simulink model "PASTd_2024"  (R2024b)
settings: Solver=VariableStepAuto  StartTime=0.0  StopTime=20  RelTol=1e-3
model workspace: external: MATLAB File PASTd_2024_saveas.m (data not in the file)
values from neighbouring files (symbols this model uses):
  B_table = cmap(:,3)'    [run.m]
  d0 = 0.01    [run.m]
  G_table = cmap(:,2)'    [run.m]
  R_table = cmap(:,1)'    [run.m]
  w0 = ones(l*w,1)    [run.m]
undefined symbols (not defined in the file or in its folder): hot, intensity_max, intensity_min, l, lower_raw, magnitude, upper_raw, w
libraries: dsparch4 x9, matrix_library x1, dspsrcs4 x1
settings Model: PacingRate=10  Creator=yingwan  LastModifiedBy=keshm
settings DebuggingCC: UnderSpecifiedDimensionMsg=warning

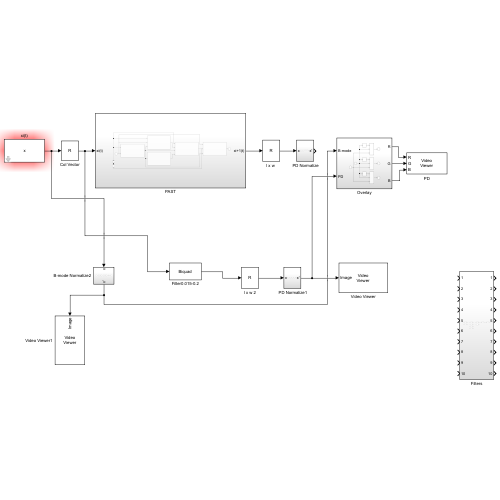
[thumbnail: Simulink's stored preview of the top-level diagram]
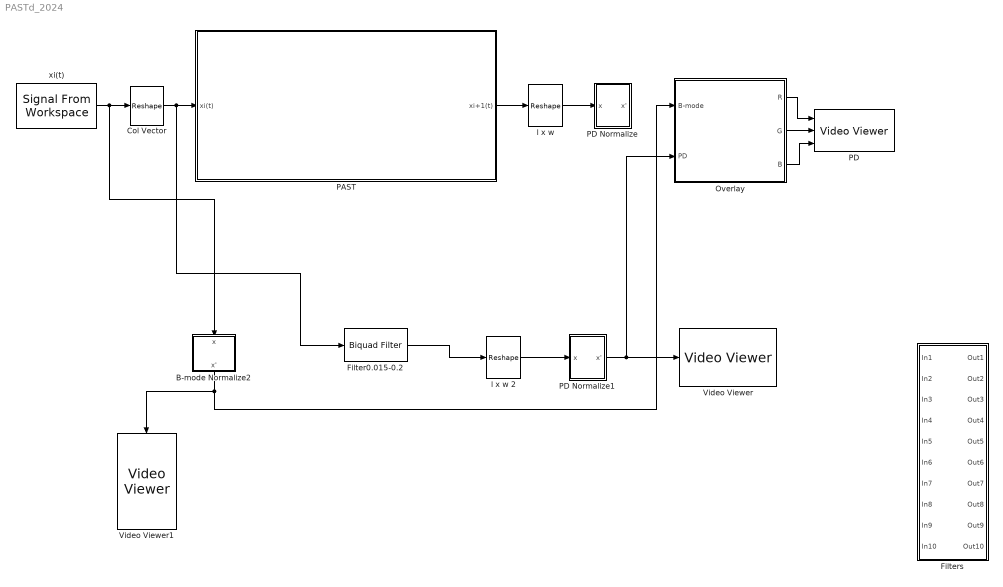
== system PASTd_2024 ==
  " PD Normalize" : Subsystem
  " PD Normalize1" : Subsystem
  B-mode Normalize2 : Subsystem
  Col Vector : Reshape  OutputDimensionality=Customize  OutputDimensions=[l*w, 1]
  Filter0.015-0.2 : dsparch4/Biquad Filter  Tag=BlockMethodSubSystem  FilterSource=Dialog parameters  CoeffSource=Specify via dialog  FilterObject=BQF  IIRFiltStruct=Direct form II  BiQuadCoeffs=[1 -2 1 1 -1.52837366682203224 0.708119014314827044;1 -2 1 1 -1.26689741225279207 0.41589168017720568]  ScaleValues=[0.809123170284214877;0.670697273107499381;1]  IC=0  ICnum=0  ICden=0  a0Flag=Warning  optimizeScaleValues=on  ScaleValueMode=Specify via input port (g)  InputProcessing=Columns as channels (frame based)  roundingMode=Floor  overflowMode=off  scaleValueFracLength=14  denProdOutputFracLength=30  denAccumFracLength=30  secondMemoryFracLength=15
  Filters : Subsystem
  Overlay : Subsystem
  PAST : Subsystem
  PD : VideoViewer  imagePorts=separate color signals  useColorMap=on  colormapValue=hot(256)  FigPos=[1.8 813.2 766.4 708]
  Video Viewer : VideoViewer  FigPos=[-11 988.4 766.4 708]
  Video Viewer1 : VideoViewer  FigPos=[139.4 813.2 766.4 708]
  "l x w " : Reshape  OutputDimensionality=Customize  OutputDimensions=[l, w]
  l x w 2 : Reshape  OutputDimensionality=Customize  OutputDimensions=[l, w]
  xi(t) : dspsrcs4/Signal From Workspace  X=x  Ts=1  nsamps=1  OutputAfterFinalValue=Setting to zero  ignoreOrWarnInputAndFrameLengths=off  OutputFrames=off
  wires:
  "l x w "/1 -> " PD Normalize"/1(x)
  Overlay/1(R) -> PD/1
  Overlay/2(G) -> PD/2
  Overlay/3(B) -> PD/3
  PAST/1(xi+1(t)) -> "l x w "/1
  l x w 2/1 -> " PD Normalize1"/1(x)
  " PD Normalize1"/1(x') -> Overlay/2(PD), Video Viewer/1
  B-mode Normalize2/1(x') -> Overlay/1(B-mode), Video Viewer1/1
  xi(t)/1 -> B-mode Normalize2/1(x), Col Vector/1
  Col Vector/1 -> Filter0.015-0.2/1, PAST/1(xi(t))
  Filter0.015-0.2/1 -> l x w 2/1

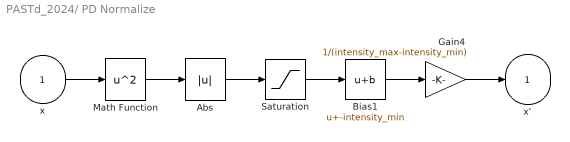
== system PASTd_2024/ PD Normalize ==
  x : Inport
  Abs : Abs  SaturateOnIntegerOverflow=off
  Bias1 : Bias  Bias=-intensity_min  SaturateOnIntegerOverflow=off
  Gain4 : Gain  Gain=1/(intensity_max-intensity_min)
  Math Function : Math  Operator=square
  Saturation : Saturate  UpperLimit=intensity_max  LowerLimit=intensity_min
  x' : Outport
  wires:
  x/1 -> Math Function/1
  Saturation/1 -> Bias1/1
  Bias1/1 -> Gain4/1
  Math Function/1 -> Abs/1
  Abs/1 -> Saturation/1
  Gain4/1 -> x'/1

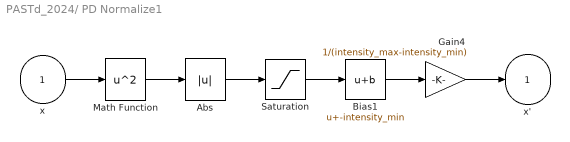
== system PASTd_2024/ PD Normalize1 ==
  x : Inport
  Abs : Abs  SaturateOnIntegerOverflow=off
  Bias1 : Bias  Bias=-intensity_min  SaturateOnIntegerOverflow=off
  Gain4 : Gain  Gain=1/(intensity_max-intensity_min)
  Math Function : Math  Operator=square
  Saturation : Saturate  UpperLimit=intensity_max  LowerLimit=intensity_min
  x' : Outport
  wires:
  x/1 -> Math Function/1
  Saturation/1 -> Bias1/1
  Bias1/1 -> Gain4/1
  Math Function/1 -> Abs/1
  Abs/1 -> Saturation/1
  Gain4/1 -> x'/1

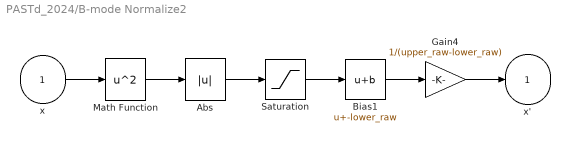
== system PASTd_2024/B-mode Normalize2 ==
  x : Inport
  Abs : Abs  SaturateOnIntegerOverflow=off
  Bias1 : Bias  Bias=-lower_raw  SaturateOnIntegerOverflow=off
  Gain4 : Gain  Gain=1/(upper_raw-lower_raw)
  Math Function : Math  Operator=square
  Saturation : Saturate  UpperLimit=upper_raw  LowerLimit=lower_raw  LinearizeAsGain=off  ZeroCross=off
  x' : Outport
  wires:
  x/1 -> Math Function/1
  Saturation/1 -> Bias1/1
  Gain4/1 -> x'/1
  Bias1/1 -> Gain4/1
  Math Function/1 -> Abs/1
  Abs/1 -> Saturation/1

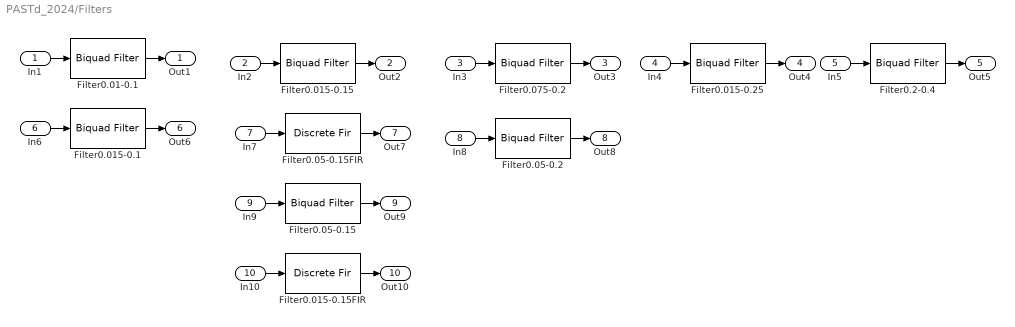
== system PASTd_2024/Filters ==
  In1 : Inport
  In2 : Inport  Port=2
  In3 : Inport  Port=3
  In4 : Inport  Port=4
  In5 : Inport  Port=5
  In6 : Inport  Port=6
  In7 : Inport  Port=7
  In8 : Inport  Port=8
  In9 : Inport  Port=9
  In10 : Inport  Port=10
  Filter0.01-0.1 : dsparch4/Biquad Filter  Tag=BlockMethodSubSystem  FilterSource=Dialog parameters  CoeffSource=Specify via dialog  FilterObject=BQF  IIRFiltStruct=Direct form II  BiQuadCoeffs=[1 -2 1 1 -1.84892349010010104 0.8856135112938337;1 -2 1 1 -1.69231556942501316 0.725897864442167084;1 -1 0 1 -0.819639680196351028 0]  ScaleValues=[0.933634250348483685;0.854553358466795032;0.909819840098175514;1]  IC=0  ICnum=0  ICden=0  a0Flag=Warning  optimizeScaleValues=on  ScaleValueMode=Specify via input port (g)  InputProcessing=Columns as channels (frame based)  roundingMode=Floor  overflowMode=off  scaleValueFracLength=14  denProdOutputFracLength=30  denAccumFracLength=30  secondMemoryFracLength=15
  Filter0.015-0.1 : dsparch4/Biquad Filter  Tag=BlockMethodSubSystem  FilterSource=Dialog parameters  CoeffSource=Specify via dialog  FilterObject=BQF  IIRFiltStruct=Direct form II  BiQuadCoeffs=[1 -2 1 1 -1.52837366682203224 0.708119014314827044;1 -2 1 1 -1.26689741225279207 0.41589168017720568]  ScaleValues=[0.809123170284214877;0.670697273107499381;1]  IC=0  ICnum=0  ICden=0  a0Flag=Warning  optimizeScaleValues=on  ScaleValueMode=Specify via input port (g)  InputProcessing=Columns as channels (frame based)  roundingMode=Floor  overflowMode=off  scaleValueFracLength=14  denProdOutputFracLength=30  denAccumFracLength=30  secondMemoryFracLength=15
  Filter0.015-0.15 : dsparch4/Biquad Filter  Tag=BlockMethodSubSystem  FilterSource=Dialog parameters  CoeffSource=Specify via dialog  FilterObject=BQF  IIRFiltStruct=Direct form II  BiQuadCoeffs=[1 -2 1 1 -1.75562644467781692 0.835014470872050274;1 -2 1 1 -1.54888704710593572 0.618926482795866928;1 -1 0 1 -0.741108729168753255 0]  ScaleValues=[0.897660228887466771;0.791953382475450662;0.870554364584376628;1]  IC=0  ICnum=0  ICden=0  a0Flag=Warning  optimizeScaleValues=on  ScaleValueMode=Specify via input port (g)  InputProcessing=Columns as channels (frame based)  roundingMode=Floor  overflowMode=off  scaleValueFracLength=14  denProdOutputFracLength=30  denAccumFracLength=30  secondMemoryFracLength=15
  Filter0.015-0.15FIR : DiscreteFir  Tag=BlockMethodSubSystem  Coefficients=[-0.00817982258423826693 -0.00115461509391236389 -0.000157645231897022512 0.00159029692229093302 0.00396257285495258457 0.00666579947044896107 0.00931195428675157463 0.0113584672677567028 0.0122257744546577767 0.0113500766030223861 0.00823512230676711268 0.00255420008832865902 -0.00579732415583847967 -0.0166526068244952051 -0.0295568789888032007 -0.0438002739207796962 -0.0584595981833108194 -0.0724821103388099408 -0.084792403945555303 -0.094398988106117715 -0.100507346913328799 0.897396592211246458 -0.100507346913328799 -0.094398988106117715 -0.084792403945555303 -0.0724821103388099408 -0.0584595981833108194 -0.0438002739207796962 -0.0295568789888032007 -0.0166526068244952051 -0.00579732415583847967 0.00255420008832865902 0.00823512230676711268 0.0113500766030223861 0.0122257744546577767 0.0113584672677567028 0.00931195428675157463 0.00666579947044896107 0.00396257285495258457 0.00159029692229093302 -0.000157645231897022512 -0.00115461509391236389 -0.00817982258423826693]  InputProcessing=Columns as channels (frame based)
  Filter0.015-0.25 : dsparch4/Biquad Filter  Tag=BlockMethodSubSystem  FilterSource=Dialog parameters  CoeffSource=Specify via dialog  FilterObject=BQF  IIRFiltStruct=Direct form II  BiQuadCoeffs=[1 -2 1 1 -1.52837366682203224 0.708119014314827044;1 -2 1 1 -1.26689741225279207 0.41589168017720568]  ScaleValues=[0.809123170284214877;0.670697273107499381;1]  IC=0  ICnum=0  ICden=0  a0Flag=Warning  optimizeScaleValues=on  ScaleValueMode=Specify via input port (g)  InputProcessing=Columns as channels (frame based)  roundingMode=Floor  overflowMode=off  scaleValueFracLength=14  denProdOutputFracLength=30  denAccumFracLength=30  secondMemoryFracLength=15
  Filter0.05-0.15 : dsparch4/Biquad Filter  Tag=BlockMethodSubSystem  FilterSource=Dialog parameters  CoeffSource=Specify via dialog  FilterObject=BQF  IIRFiltStruct=Direct form II  BiQuadCoeffs=[1 -2 1 1 -1.69400644668283573 0.864672027053842274;1 -2 1 1 -1.50288901397170971 0.65430014130534353;1 -2 1 1 -1.37630787767555174 0.514966371669266398;1 -2 1 1 -1.30458925897473432 0.436022337912945812;1 -1 0 1 -0.640699622503299704 0]  ScaleValues=[0.889669618434169474;0.78929728881926331;0.722818562336204562;0.68515289922192002;0.820349811251649852;1]  IC=0  ICnum=0  ICden=0  a0Flag=Warning  optimizeScaleValues=on  ScaleValueMode=Specify via input port (g)  InputProcessing=Columns as channels (frame based)  roundingMode=Floor  overflowMode=off  scaleValueFracLength=14  denProdOutputFracLength=30  denAccumFracLength=30  secondMemoryFracLength=15
  Filter0.05-0.15FIR : DiscreteFir  Tag=BlockMethodSubSystem  Coefficients=[-0.00429721268483966232 0.0104011527547215182 0.00305322596265845091 -0.000165202304057802626 -0.00216746345798422314 -0.00387292162250563437 -0.00534681034917153675 -0.00637393415041462037 -0.00658426761661669215 -0.00568806394226628858 -0.00351624416374436829 -7.34566575591197806e-05 0.00435696609728229104 0.00926947324682613275 0.0139530342143546534 0.0175380630724172246 0.0191189672514937119 0.0178725969589094112 0.013187761673555759 0.00475230538552628718 -0.00736052606321290284 -0.0226334065737471037 -0.0401484008223075145 -0.0586623112683273343 -0.076714250024829983 -0.0927775538057464128 -0.105428635000339513 -0.113519726534417081 0.883695812069324682 -0.113519726534417081 -0.105428635000339513 -0.0927775538057464128 -0.076714250024829983 -0.0586623112683273343 -0.0401484008223075145 -0.0226334065737471037 -0.00736052606321290284 0.00475230538552628718 0.013187761673555759 0.0178725969589094112 0.0191189672514937119 0.0175380630724172246 0.0139530342143546534 0.00926947324682613275 0.00435696609728229104 -7.34566575591197806e-05 -0.00351624416374436829 -0.00568806394226628858 -0.00658426761661669215 -0.00637393415041462037 -0.00534681034917153675 -0.00387292162250563437 -0.00216746345798422314 -0.000165202304057802626 0.00305322596265845091 0.0104011527547215182 -0.00429721268483966232]  InputProcessing=Columns as channels (frame based)
  Filter0.05-0.2 : dsparch4/Biquad Filter  Tag=BlockMethodSubSystem  FilterSource=Dialog parameters  CoeffSource=Specify via dialog  FilterObject=BQF  IIRFiltStruct=Direct form II  BiQuadCoeffs=[1 -2 1 1 -1.50240971938457935 0.785371909972968019;1 -2 1 1 -1.25896047022456226 0.496071697556646651;1 -2 1 1 -1.13202167631421302 0.345225391113541724;1 -1 0 1 -0.54635031844578863 0]  ScaleValues=[0.821945407339386813;0.688758041945302213;0.619311766856938672;0.77317515922289437;1]  IC=0  ICnum=0  ICden=0  a0Flag=Warning  optimizeScaleValues=on  ScaleValueMode=Specify via input port (g)  InputProcessing=Columns as channels (frame based)  roundingMode=Floor  overflowMode=off  scaleValueFracLength=14  denProdOutputFracLength=30  denAccumFracLength=30  secondMemoryFracLength=15
  Filter0.075-0.2 : dsparch4/Biquad Filter  Tag=BlockMethodSubSystem  FilterSource=Dialog parameters  CoeffSource=Specify via dialog  FilterObject=BQF  IIRFiltStruct=Direct form II  BiQuadCoeffs=[1 -2 1 1 -1.54326811238169803 0.842532579516595992;1 -2 1 1 -1.34225190781423809 0.602536105180896397;1 -2 1 1 -1.20836471381479216 0.442686034448000143;1 -2 1 1 -1.12671053673786825 0.345197801320664743;1 -2 1 1 -1.0880564447293537 0.299048060205749089]  ScaleValues=[0.846450172974573589;0.736197003248783566;0.662762687065698075;0.61797708451463329;0.596776126233775739;1]  IC=0  ICnum=0  ICden=0  a0Flag=Warning  optimizeScaleValues=on  ScaleValueMode=Specify via input port (g)  InputProcessing=Columns as channels (frame based)  roundingMode=Floor  overflowMode=off  scaleValueFracLength=14  denProdOutputFracLength=30  denAccumFracLength=30  secondMemoryFracLength=15
  Filter0.2-0.4 : dsparch4/Biquad Filter  Tag=BlockMethodSubSystem  FilterSource=Dialog parameters  CoeffSource=Specify via dialog  FilterObject=BQF  IIRFiltStruct=Direct form II  BiQuadCoeffs=[1 -2 1 1 -1.150551993440043 0.892780982171610615;1 -2 1 1 -1.04016200959971727 0.711177662003108835;1 -2 1 1 -0.951653092896676989 0.56557103558092281;1 -2 1 1 -0.880614280792255233 0.448704598154408607;1 -2 1 1 -0.823745826054325114 0.355149912901455422;1 -2 1 1 -0.778577051080206473 0.280842451138358651;1 -2 1 1 -0.743262138541350592 0.222745646107631978;1 -2 1 1 -0.716433877054854285 0.178610288978277132;1 -2 1 1 -0.697099999701282003 0.146803994629887913;1 -2 1 1 -0.684571005858506498 0.126192460856045852;1 -2 1 1 -0.678411758768196926 0.116059841188700857]  ScaleValues=[0.760833243902913403;0.6878349179007065;0.62930603211939995;0.582329719736665918;0.544723934738945204;0.514854875554641267;0.491501946162245629;0.473761041508282854;0.460975998582792479;0.452690866678638115;0.448617899989224467;1]  IC=0  ICnum=0  ICden=0  a0Flag=Warning  optimizeScaleValues=on  ScaleValueMode=Specify via input port (g)  InputProcessing=Columns as channels (frame based)  roundingMode=Floor  overflowMode=off  scaleValueFracLength=14  denProdOutputFracLength=30  denAccumFracLength=30  secondMemoryFracLength=15
  Out1 : Outport
  Out2 : Outport  Port=2
  Out3 : Outport  Port=3
  Out4 : Outport  Port=4
  Out5 : Outport  Port=5
  Out6 : Outport  Port=6
  Out7 : Outport  Port=7
  Out8 : Outport  Port=8
  Out9 : Outport  Port=9
  Out10 : Outport  Port=10
  wires:
  In10/1 -> Filter0.015-0.15FIR/1
  Filter0.2-0.4/1 -> Out5/1
  In2/1 -> Filter0.015-0.15/1
  Filter0.015-0.25/1 -> Out4/1
  Filter0.05-0.2/1 -> Out8/1
  In4/1 -> Filter0.015-0.25/1
  In3/1 -> Filter0.075-0.2/1
  In8/1 -> Filter0.05-0.2/1
  Filter0.05-0.15FIR/1 -> Out7/1
  In6/1 -> Filter0.015-0.1/1
  Filter0.015-0.15FIR/1 -> Out10/1
  Filter0.075-0.2/1 -> Out3/1
  In7/1 -> Filter0.05-0.15FIR/1
  Filter0.01-0.1/1 -> Out1/1
  Filter0.015-0.15/1 -> Out2/1
  Filter0.05-0.15/1 -> Out9/1
  In1/1 -> Filter0.01-0.1/1
  Filter0.015-0.1/1 -> Out6/1
  In9/1 -> Filter0.05-0.15/1
  In5/1 -> Filter0.2-0.4/1

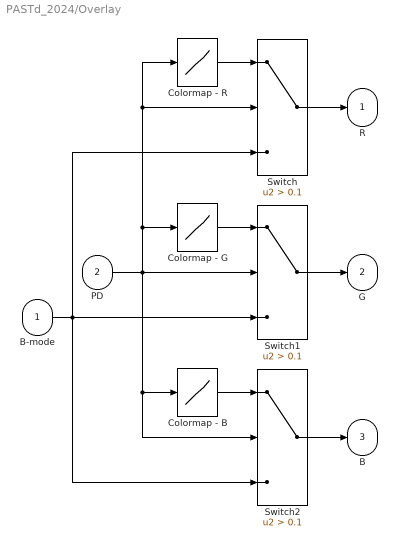
== system PASTd_2024/Overlay ==
  B-mode : Inport
  PD : Inport  Port=2
  Colormap - B : Lookup_n-D  NumberOfTableDimensions=1  BreakpointsForDimension1=linspace(0,255,256)  Table=B_table * 255  InternalRulePriority=Speed  RndMeth=Simplest
  Colormap - G : Lookup_n-D  NumberOfTableDimensions=1  BreakpointsForDimension1=linspace(0,255,256)  Table=G_table * 255  InternalRulePriority=Speed  RndMeth=Simplest
  Colormap - R : Lookup_n-D  NumberOfTableDimensions=1  BreakpointsForDimension1=linspace(0,255,256)  Table=R_table * 255  InternalRulePriority=Speed  RndMeth=Simplest
  Switch : Switch  Criteria=u2 > Threshold  Threshold=0.1  SaturateOnIntegerOverflow=off  InputSameDT=off
  Switch1 : Switch  Criteria=u2 > Threshold  Threshold=0.1  SaturateOnIntegerOverflow=off  InputSameDT=off
  Switch2 : Switch  Criteria=u2 > Threshold  Threshold=0.1  SaturateOnIntegerOverflow=off  InputSameDT=off
  R : Outport
  G : Outport  Port=2
  B : Outport  Port=3
  wires:
  PD/1 -> Switch2/2, Colormap - B/1, Colormap - R/1, Switch/2, Colormap - G/1, Switch1/2
  Colormap - R/1 -> Switch/1
  B-mode/1 -> Switch2/3, Switch/3, Switch1/3
  Colormap - G/1 -> Switch1/1
  Colormap - B/1 -> Switch2/1
  Switch1/1 -> G/1
  Switch/1 -> R/1
  Switch2/1 -> B/1

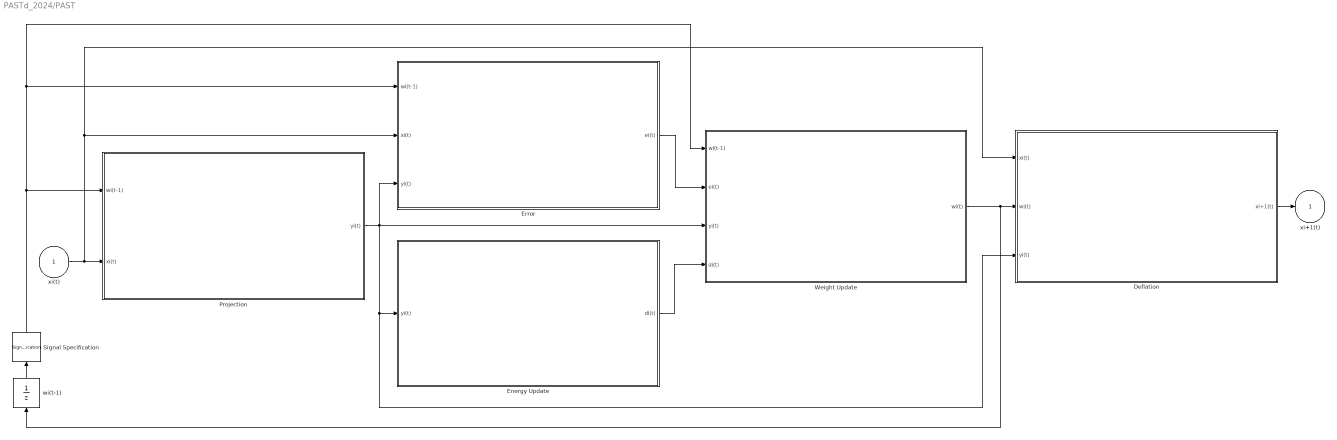
== system PASTd_2024/PAST ==
  xi(t) : Inport  PortDimensions=[l*w, 1]
  " Deflation" : Subsystem
  " Weight Update" : Subsystem
  "Energy Update  " : Subsystem
  "Error   " : Subsystem
  Projection : Subsystem
  Signal Specification : SignalSpecification  Dimensions=[l*w, 1]
  "wi(t-1) " : UnitDelay  InitialCondition=w0  SampleTime=-1  HasFrameUpgradeWarning=on
  xi+1(t) : Outport
  wires:
  " Deflation"/1(xi+1(t)) -> xi+1(t)/1
  "Error   "/1(ei(t)) -> " Weight Update"/2(ei(t))
  " Weight Update"/1(wi(t)) -> "wi(t-1) "/1, " Deflation"/2(wi(t))
  Projection/1(yi(t)) -> "Error   "/3(yi(t)), " Weight Update"/3(yi(t)), " Deflation"/3(yi(t)), "Energy Update  "/1(yi(t))
  xi(t)/1 -> Projection/2(xi(t)), "Error   "/2(xi(t)), " Deflation"/1(xi(t))
  "wi(t-1) "/1 -> Signal Specification/1
  Signal Specification/1 -> Projection/1(wi(t-1)), " Weight Update"/1(wi(t-1)), "Error   "/1(wi(t-1))
  "Energy Update  "/1(di(t)) -> " Weight Update"/4(di(t))

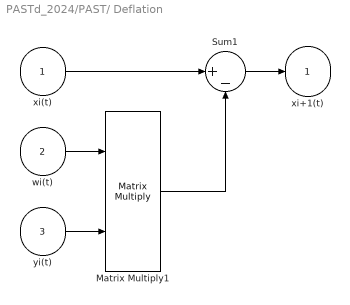
== system PASTd_2024/PAST/ Deflation ==
  xi(t) : Inport  PortDimensions=[l*w, 1]
  wi(t) : Inport  Port=2  PortDimensions=[l*w, 1]
  yi(t) : Inport  Port=3  PortDimensions=[1,1]
  Matrix Multiply1 : Product  Multiplication=Matrix(*)
  Sum1 : Sum  Inputs=|+-
  xi+1(t) : Outport  PortDimensions=[l*w, 1]
  wires:
  xi(t)/1 -> Sum1/1
  Sum1/1 -> xi+1(t)/1
  Matrix Multiply1/1 -> Sum1/2
  wi(t)/1 -> Matrix Multiply1/1
  yi(t)/1 -> Matrix Multiply1/2

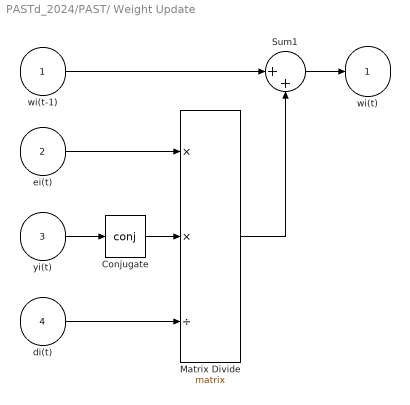
== system PASTd_2024/PAST/ Weight Update ==
  wi(t-1) : Inport  PortDimensions=[l*w, 1]
  ei(t) : Inport  Port=2  PortDimensions=[l*w, 1]
  yi(t) : Inport  Port=3  PortDimensions=[1,1]
  di(t) : Inport  Port=4  PortDimensions=[1,1]
  Conjugate : Math  Operator=conj  SignedPower=on  RndMeth=Zero
  Matrix Divide : Product  Inputs=**/  Multiplication=Matrix(*)
  Sum1 : Sum  Inputs=|++
  wi(t) : Outport  PortDimensions=[l*w, 1]
  wires:
  yi(t)/1 -> Conjugate/1
  di(t)/1 -> Matrix Divide/3
  wi(t-1)/1 -> Sum1/1
  Matrix Divide/1 -> Sum1/2
  Sum1/1 -> wi(t)/1
  Conjugate/1 -> Matrix Divide/2
  ei(t)/1 -> Matrix Divide/1

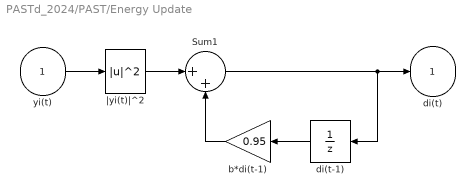
== system PASTd_2024/PAST/Energy Update   ==
  yi(t) : Inport  PortDimensions=[1,1]
  Sum1 : Sum  Inputs=|++
  b*di(t-1) : Gain  Gain=0.95
  di(t-1) : UnitDelay  InitialCondition=d0  SampleTime=-1  HasFrameUpgradeWarning=on
  |yi(t)|^2 : Math  Operator=magnitude^2
  di(t) : Outport  PortDimensions=[1,1]
  wires:
  b*di(t-1)/1 -> Sum1/2
  yi(t)/1 -> |yi(t)|^2/1
  |yi(t)|^2/1 -> Sum1/1
  di(t-1)/1 -> b*di(t-1)/1
  Sum1/1 -> di(t-1)/1, di(t)/1

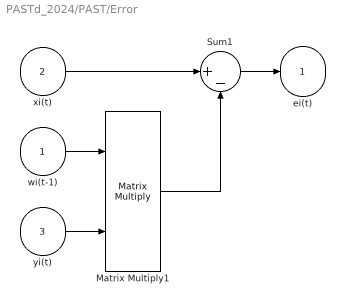
== system PASTd_2024/PAST/Error    ==
  wi(t-1) : Inport  PortDimensions=[l*w, 1]
  xi(t) : Inport  Port=2
  yi(t) : Inport  Port=3  PortDimensions=[1,1]
  Matrix Multiply1 : Product  Multiplication=Matrix(*)
  Sum1 : Sum  Inputs=|+-
  ei(t) : Outport  PortDimensions=[l*w, 1]
  wires:
  Matrix Multiply1/1 -> Sum1/2
  Sum1/1 -> ei(t)/1
  xi(t)/1 -> Sum1/1
  wi(t-1)/1 -> Matrix Multiply1/1
  yi(t)/1 -> Matrix Multiply1/2

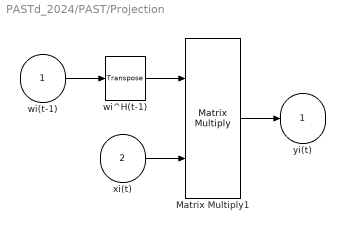
== system PASTd_2024/PAST/Projection ==
  wi(t-1) : Inport  PortDimensions=[l*w, 1]
  xi(t) : Inport  Port=2  PortDimensions=[l*w, 1]
  Matrix Multiply1 : Product  Multiplication=Matrix(*)
  wi^H(t-1) : matrix_library/Transpose
  yi(t) : Outport  PortDimensions=[1,1]
  wires:
  wi(t-1)/1 -> wi^H(t-1)/1
  xi(t)/1 -> Matrix Multiply1/2
  wi^H(t-1)/1 -> Matrix Multiply1/1
  Matrix Multiply1/1 -> yi(t)/1
